simulink model "For_inv"  (R2021a)
settings: Solver=VariableStepAuto  StartTime=0.0  StopTime=10  MaxStep=0.001  RelTol=1e-3
model workspace: external: MATLAB File C:\Users\ACER\Downloads\try8\try8_DataFile.m (data not in the file)
values from neighbouring files (symbols this model uses):
  X = [X; end_effector_pos']    [generate_dataset.m]
undefined symbols (not defined in the file or in its folder): NBits, smiData, Y, Z
libraries: sm_lib x146, nesl_utility x9, robotmaniplib x2, robotcorelib x1, msbAdcArchitectures x1, deeplib x1, simulink x1
(part 1 of 4)
settings Model: Creator=ACER  LastModifiedBy=user

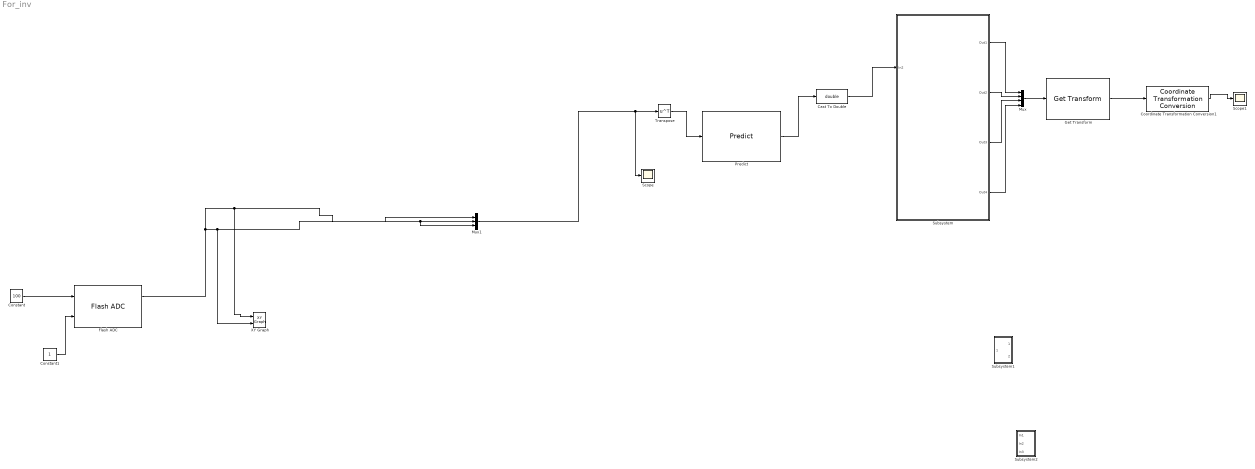
== system For_inv ==
  Cast To Double : DataTypeConversion  OutDataTypeStr=double
  Constant : Constant  Value=100
  Constant1 : Constant
  Coordinate Transformation Conversion1 : robotcorelib/Coordinate Transformation Conversion  InputRepresentation=Homogeneous Transformation  InputEulerSequence=ZYX  ShowTrVecInputPort=on  OutputRepresentation=Translation Vector  OutputEulerSequence=ZYX  ShowTrVecOutputPort=on  SimulateUsing=Interpreted execution
      settings: SourceProductBaseCode=NV,RO,RR,UV
  Flash ADC : msbAdcArchitectures/Flash ADC  NBits=10  InputRange=[-1 1]  ExtStartClk=on  StartFreq=1e6  StartClkJitter=1e-12  Trigger=Rising edge  MatchScale=off  OutputPolarity=Auto  OutDataType=fixdt(1,NBits)  EnableImp=off  OffsetError=3  OffsetErrorUnit=LSB  GainError=2  GainErrorUnit=LSB  Bubbles=[]
      settings: SourceProductBaseCode=AM
  Get Transform : robotmaniplib/Get Transform  RigidBodyTree=Modelrobot  SourceBody=base_link  TargetBody=wrist  SimulateUsing=Interpreted execution
  Mux : Mux
  Mux1 : Mux  Inputs=3
  Predict : deeplib/Predict  Network=Network from MAT-file  NetworkFunction=squeezenet  NetworkFilePath=E:\term9\project1\neural_network_for_robot_arm\trained_network.mat  MiniBatchSize=64  InputDataFormats={ '', '' }  Predictions=on  Activations={}  ForceInterpretedSim=off  EnableDLNetwork=on
      link override "MLFB/ Demux ": Outputs=1
      link override MLFB/in_1: Port=1
      link override MLFB/out_1_predict: Port=1
      settings: SourceProductBaseCode=NN
  Scope : Scope
  Scope1 : Scope
  Subsystem : Subsystem
  Subsystem1 : Subsystem
  Subsystem2 : Subsystem
  Transpose : Math  Operator=transpose  SaturateOnIntegerOverflow=on
  XY Graph : simulink/Sinks/XY Graph  xmin=0  xmax=350  ymin=0  ymax=350  st=-1
  wires:
  Get Transform/1 -> Coordinate Transformation Conversion1/1
  Mux/1 -> Get Transform/1
  Subsystem/1(Out1) -> Mux/1
  Subsystem/2(Out2) -> Mux/2
  Subsystem/3(Out3) -> Mux/3
  Subsystem/4(Out4) -> Mux/4
  Coordinate Transformation Conversion1/1 -> Scope1/1
  Transpose/1 -> Predict/1
  Predict/1 -> Cast To Double/1
  Cast To Double/1 -> Subsystem/1(In2)
  Mux1/1 -> Scope/1, Transpose/1
  Flash ADC/1 -> XY Graph/1, Mux1/1, XY Graph/2, Mux1/3, Mux1/2
  Constant/1 -> Flash ADC/1
  Constant1/1 -> Flash ADC/2
